simulink model "AUV_velocity_controller"  (R2020b)
settings: Solver=VariableStepAuto  StartTime=0.0  StopTime=400  RelTol=1e-3
libraries: pid_lib x16, robotcorelib x1, dspsigops x1
(part 2 of 2)

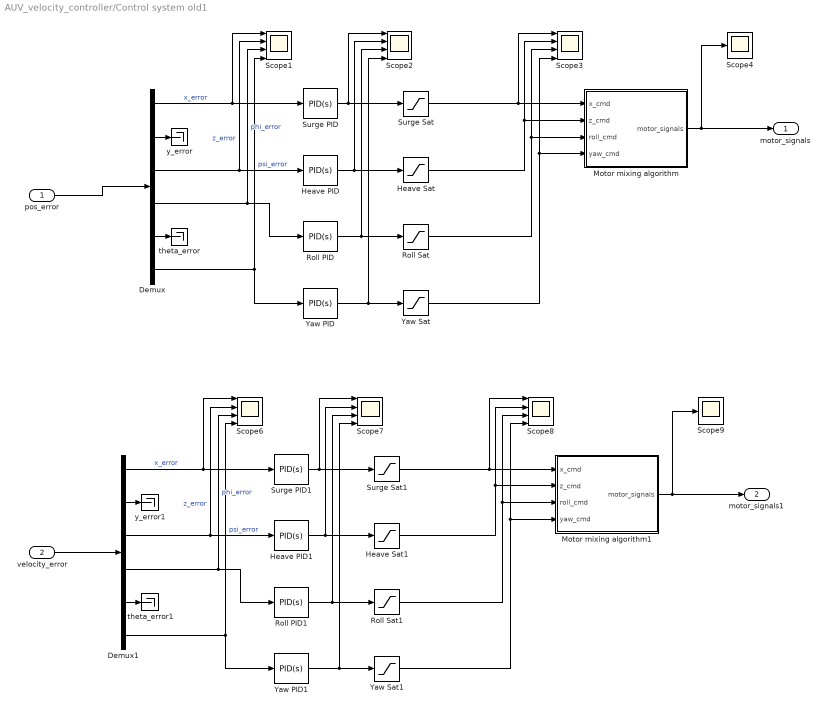
== system AUV_velocity_controller/Control system old1 ==
  pos_error : Inport
  velocity_error : Inport  Port=2
  Demux : Demux  Outputs=6
  Demux1 : Demux  Outputs=6
  Heave PID : pid_lib/PID Controller  Controller=PID  Form=Parallel  TimeDomain=Continuous-time  UseExternalTs=off  SampleTime=-1  IntegratorMethod=Forward Euler  FilterMethod=Forward Euler  ControllerParametersSource=internal  P=5  I=0  D=2  UseFilter=on  N=100  TunerSelectOption=Transfer Function Based (PID Tuner App)  InitialConditionSource=internal  InitialConditionForIntegrator=0  InitialConditionForFilter=0  DifferentiatorICPrevScaledInput=0  ExternalReset=none  TrackingMode=off  Kt=1  LimitOutput=on  SatLimitsSource=internal  UpperSaturationLimit=10  LowerSaturationLimit=-10  LinearizeAsGain=on  AntiWindupMode=clamping  Kb=1  POutMin=[]  POutMax=[]  IOutMin=[]  IOutMax=[]  DOutMin=[]  DOutMax=[]  NOutMin=[]  NOutMax=[]  SumOutMin=[]  SumOutMax=[]  SaturationOutMin=[]  SaturationOutMax=[]  PParamMin=[]  PParamMax=[]  IParamMin=[]  IParamMax=[]  DParamMin=[]  DParamMax=[]  NParamMin=[]  NParamMax=[]  KbParamMin=[]  KbParamMax=[]  KtParamMin=[]  KtParamMax=[]  KbOutMin=[]  KbOutMax=[]  KtOutMin=[]  KtOutMax=[]  IntegratorOutMin=[]  IntegratorOutMax=[]  FilterOutMin=[]  FilterOutMax=[]  SumI1OutMin=[]  SumI1OutMax=[]  SumI2OutMin=[]  SumI2OutMax=[]  SumI3OutMin=[]  SumI3OutMax=[]  SumI4OutMin=[]  SumI4OutMax=[]  SumDOutMin=[]  SumDOutMax=[]  DifferentiatorOutMin=[]  DifferentiatorOutMax=[]  FilterDiffOutCoefMin=[]  FilterDiffOutCoefMax=[]  ReciprocalOutMin=[]  ReciprocalOutMax=[]  SumDenOutMin=[]  SumDenOutMax=[]  SumNumOutMin=[]  SumNumOutMax=[]  DivideOutMin=[]  DivideOutMax=[]  UdiffTsProdOutMin=[]  UdiffTsProdOutMax=[]  NTsProdOutMin=[]  NTsProdOutMax=[]  UintegralTsProdOutMin=[]  UintegralTsProdOutMax=[]  UngainTsProdOutMin=[]  UngainTsProdOutMax=[]  IntegratorContinuousStateAttributes=''  IntegratorStateMustResolveToSignalObject=off  IntegratorRTWStateStorageClass=Auto  FilterContinuousStateAttributes=''  FilterStateMustResolveToSignalObject=off  FilterRTWStateStorageClass=Auto  ParallelPVariant=InternalParameters  IdealPVariant=Disabled  IVariant=InternalParameters  DVariant=InternalParameters  IntegratorVariant=Continuous  SatVariant=Enabled  AWVariant=ContClampingParallel  PCopyVariant=Disabled  TRVariant=Disabled  FdbkBlocksVariant=Forward  IdealPFdbkVariant=Disabled  SatFdbkVariant=Disabled  DerivativeFilterVariant=ContFilter  NVariant=InternalParameters  NCopyVariant=Disabled  FilterICVariant=InternalICsFilter  IntegratorICVariant=InternalICs  ExternalResetVariant=Disabled  TRSumVariant=Passthrough  SumFdbkVariant=Disabled  SumVariant=Sum_PID  TsampFilterVariant=InternalTs  TsampNgainVariant=Passthrough  TsampIntegralVariant=Passthrough  ExternalSaturationOutDataTypeStr=Inherit: Same as second input
  Heave PID1 : pid_lib/PID Controller  Controller=PID  Form=Parallel  TimeDomain=Continuous-time  UseExternalTs=off  SampleTime=-1  IntegratorMethod=Forward Euler  FilterMethod=Forward Euler  ControllerParametersSource=internal  P=5  I=0  D=2  UseFilter=on  N=100  TunerSelectOption=Transfer Function Based (PID Tuner App)  InitialConditionSource=internal  InitialConditionForIntegrator=0  InitialConditionForFilter=0  DifferentiatorICPrevScaledInput=0  ExternalReset=none  TrackingMode=off  Kt=1  LimitOutput=on  SatLimitsSource=internal  UpperSaturationLimit=10  LowerSaturationLimit=-10  LinearizeAsGain=on  AntiWindupMode=clamping  Kb=1  POutMin=[]  POutMax=[]  IOutMin=[]  IOutMax=[]  DOutMin=[]  DOutMax=[]  NOutMin=[]  NOutMax=[]  SumOutMin=[]  SumOutMax=[]  SaturationOutMin=[]  SaturationOutMax=[]  PParamMin=[]  PParamMax=[]  IParamMin=[]  IParamMax=[]  DParamMin=[]  DParamMax=[]  NParamMin=[]  NParamMax=[]  KbParamMin=[]  KbParamMax=[]  KtParamMin=[]  KtParamMax=[]  KbOutMin=[]  KbOutMax=[]  KtOutMin=[]  KtOutMax=[]  IntegratorOutMin=[]  IntegratorOutMax=[]  FilterOutMin=[]  FilterOutMax=[]  SumI1OutMin=[]  SumI1OutMax=[]  SumI2OutMin=[]  SumI2OutMax=[]  SumI3OutMin=[]  SumI3OutMax=[]  SumI4OutMin=[]  SumI4OutMax=[]  SumDOutMin=[]  SumDOutMax=[]  DifferentiatorOutMin=[]  DifferentiatorOutMax=[]  FilterDiffOutCoefMin=[]  FilterDiffOutCoefMax=[]  ReciprocalOutMin=[]  ReciprocalOutMax=[]  SumDenOutMin=[]  SumDenOutMax=[]  SumNumOutMin=[]  SumNumOutMax=[]  DivideOutMin=[]  DivideOutMax=[]  UdiffTsProdOutMin=[]  UdiffTsProdOutMax=[]  NTsProdOutMin=[]  NTsProdOutMax=[]  UintegralTsProdOutMin=[]  UintegralTsProdOutMax=[]  UngainTsProdOutMin=[]  UngainTsProdOutMax=[]  IntegratorContinuousStateAttributes=''  IntegratorStateMustResolveToSignalObject=off  IntegratorRTWStateStorageClass=Auto  FilterContinuousStateAttributes=''  FilterStateMustResolveToSignalObject=off  FilterRTWStateStorageClass=Auto  ParallelPVariant=InternalParameters  IdealPVariant=Disabled  IVariant=InternalParameters  DVariant=InternalParameters  IntegratorVariant=Continuous  SatVariant=Enabled  AWVariant=ContClampingParallel  PCopyVariant=Disabled  TRVariant=Disabled  FdbkBlocksVariant=Forward  IdealPFdbkVariant=Disabled  SatFdbkVariant=Disabled  DerivativeFilterVariant=ContFilter  NVariant=InternalParameters  NCopyVariant=Disabled  FilterICVariant=InternalICsFilter  IntegratorICVariant=InternalICs  ExternalResetVariant=Disabled  TRSumVariant=Passthrough  SumFdbkVariant=Disabled  SumVariant=Sum_PID  TsampFilterVariant=InternalTs  TsampNgainVariant=Passthrough  TsampIntegralVariant=Passthrough  ExternalSaturationOutDataTypeStr=Inherit: Same as second input
  Heave Sat : Saturate  UpperLimit=10  LowerLimit=-10  ZeroCross=off
  Heave Sat1 : Saturate  UpperLimit=10  LowerLimit=-10  ZeroCross=off
  Motor mixing algorithm : MATLAB Function  TreatAsAtomicUnit=on
  Motor mixing algorithm1 : MATLAB Function  TreatAsAtomicUnit=on
  Roll PID : pid_lib/PID Controller  Controller=PID  Form=Parallel  TimeDomain=Continuous-time  UseExternalTs=off  SampleTime=-1  IntegratorMethod=Forward Euler  FilterMethod=Forward Euler  ControllerParametersSource=internal  P=5  I=0  D=2  UseFilter=on  N=100  TunerSelectOption=Transfer Function Based (PID Tuner App)  InitialConditionSource=internal  InitialConditionForIntegrator=0  InitialConditionForFilter=0  DifferentiatorICPrevScaledInput=0  ExternalReset=none  TrackingMode=off  Kt=1  LimitOutput=off  SatLimitsSource=internal  UpperSaturationLimit=inf  LowerSaturationLimit=-inf  LinearizeAsGain=on  AntiWindupMode=none  Kb=1  POutMin=[]  POutMax=[]  IOutMin=[]  IOutMax=[]  DOutMin=[]  DOutMax=[]  NOutMin=[]  NOutMax=[]  SumOutMin=[]  SumOutMax=[]  SaturationOutMin=[]  SaturationOutMax=[]  PParamMin=[]  PParamMax=[]  IParamMin=[]  IParamMax=[]  DParamMin=[]  DParamMax=[]  NParamMin=[]  NParamMax=[]  KbParamMin=[]  KbParamMax=[]  KtParamMin=[]  KtParamMax=[]  KbOutMin=[]  KbOutMax=[]  KtOutMin=[]  KtOutMax=[]  IntegratorOutMin=[]  IntegratorOutMax=[]  FilterOutMin=[]  FilterOutMax=[]  SumI1OutMin=[]  SumI1OutMax=[]  SumI2OutMin=[]  SumI2OutMax=[]  SumI3OutMin=[]  SumI3OutMax=[]  SumI4OutMin=[]  SumI4OutMax=[]  SumDOutMin=[]  SumDOutMax=[]  DifferentiatorOutMin=[]  DifferentiatorOutMax=[]  FilterDiffOutCoefMin=[]  FilterDiffOutCoefMax=[]  ReciprocalOutMin=[]  ReciprocalOutMax=[]  SumDenOutMin=[]  SumDenOutMax=[]  SumNumOutMin=[]  SumNumOutMax=[]  DivideOutMin=[]  DivideOutMax=[]  UdiffTsProdOutMin=[]  UdiffTsProdOutMax=[]  NTsProdOutMin=[]  NTsProdOutMax=[]  UintegralTsProdOutMin=[]  UintegralTsProdOutMax=[]  UngainTsProdOutMin=[]  UngainTsProdOutMax=[]  IntegratorContinuousStateAttributes=''  IntegratorStateMustResolveToSignalObject=off  IntegratorRTWStateStorageClass=Auto  FilterContinuousStateAttributes=''  FilterStateMustResolveToSignalObject=off  FilterRTWStateStorageClass=Auto  ParallelPVariant=InternalParameters  IdealPVariant=Disabled  IVariant=InternalParameters  DVariant=InternalParameters  IntegratorVariant=Continuous  SatVariant=Disabled  AWVariant=Passthrough  PCopyVariant=Disabled  TRVariant=Disabled  FdbkBlocksVariant=Forward  IdealPFdbkVariant=Disabled  SatFdbkVariant=Disabled  DerivativeFilterVariant=ContFilter  NVariant=InternalParameters  NCopyVariant=Disabled  FilterICVariant=InternalICsFilter  IntegratorICVariant=InternalICs  ExternalResetVariant=Disabled  TRSumVariant=Passthrough  SumFdbkVariant=Disabled  SumVariant=Sum_PID  TsampFilterVariant=InternalTs  TsampNgainVariant=Passthrough  TsampIntegralVariant=Passthrough  ExternalSaturationOutDataTypeStr=Inherit: Same as second input
  Roll PID1 : pid_lib/PID Controller  Controller=PID  Form=Parallel  TimeDomain=Continuous-time  UseExternalTs=off  SampleTime=-1  IntegratorMethod=Forward Euler  FilterMethod=Forward Euler  ControllerParametersSource=internal  P=5  I=0  D=2  UseFilter=on  N=100  TunerSelectOption=Transfer Function Based (PID Tuner App)  InitialConditionSource=internal  InitialConditionForIntegrator=0  InitialConditionForFilter=0  DifferentiatorICPrevScaledInput=0  ExternalReset=none  TrackingMode=off  Kt=1  LimitOutput=off  SatLimitsSource=internal  UpperSaturationLimit=inf  LowerSaturationLimit=-inf  LinearizeAsGain=on  AntiWindupMode=none  Kb=1  POutMin=[]  POutMax=[]  IOutMin=[]  IOutMax=[]  DOutMin=[]  DOutMax=[]  NOutMin=[]  NOutMax=[]  SumOutMin=[]  SumOutMax=[]  SaturationOutMin=[]  SaturationOutMax=[]  PParamMin=[]  PParamMax=[]  IParamMin=[]  IParamMax=[]  DParamMin=[]  DParamMax=[]  NParamMin=[]  NParamMax=[]  KbParamMin=[]  KbParamMax=[]  KtParamMin=[]  KtParamMax=[]  KbOutMin=[]  KbOutMax=[]  KtOutMin=[]  KtOutMax=[]  IntegratorOutMin=[]  IntegratorOutMax=[]  FilterOutMin=[]  FilterOutMax=[]  SumI1OutMin=[]  SumI1OutMax=[]  SumI2OutMin=[]  SumI2OutMax=[]  SumI3OutMin=[]  SumI3OutMax=[]  SumI4OutMin=[]  SumI4OutMax=[]  SumDOutMin=[]  SumDOutMax=[]  DifferentiatorOutMin=[]  DifferentiatorOutMax=[]  FilterDiffOutCoefMin=[]  FilterDiffOutCoefMax=[]  ReciprocalOutMin=[]  ReciprocalOutMax=[]  SumDenOutMin=[]  SumDenOutMax=[]  SumNumOutMin=[]  SumNumOutMax=[]  DivideOutMin=[]  DivideOutMax=[]  UdiffTsProdOutMin=[]  UdiffTsProdOutMax=[]  NTsProdOutMin=[]  NTsProdOutMax=[]  UintegralTsProdOutMin=[]  UintegralTsProdOutMax=[]  UngainTsProdOutMin=[]  UngainTsProdOutMax=[]  IntegratorContinuousStateAttributes=''  IntegratorStateMustResolveToSignalObject=off  IntegratorRTWStateStorageClass=Auto  FilterContinuousStateAttributes=''  FilterStateMustResolveToSignalObject=off  FilterRTWStateStorageClass=Auto  ParallelPVariant=InternalParameters  IdealPVariant=Disabled  IVariant=InternalParameters  DVariant=InternalParameters  IntegratorVariant=Continuous  SatVariant=Disabled  AWVariant=Passthrough  PCopyVariant=Disabled  TRVariant=Disabled  FdbkBlocksVariant=Forward  IdealPFdbkVariant=Disabled  SatFdbkVariant=Disabled  DerivativeFilterVariant=ContFilter  NVariant=InternalParameters  NCopyVariant=Disabled  FilterICVariant=InternalICsFilter  IntegratorICVariant=InternalICs  ExternalResetVariant=Disabled  TRSumVariant=Passthrough  SumFdbkVariant=Disabled  SumVariant=Sum_PID  TsampFilterVariant=InternalTs  TsampNgainVariant=Passthrough  TsampIntegralVariant=Passthrough  ExternalSaturationOutDataTypeStr=Inherit: Same as second input
  Roll Sat : Saturate  UpperLimit=10  LowerLimit=-10  ZeroCross=off
  Roll Sat1 : Saturate  UpperLimit=10  LowerLimit=-10  ZeroCross=off
  Scope{1..3,6..8} (6 alike) : Scope  NumInputPorts=4
  Scope4 : Scope
  Scope9 : Scope
  Surge PID : pid_lib/PID Controller  Controller=PID  Form=Parallel  TimeDomain=Continuous-time  UseExternalTs=off  SampleTime=-1  IntegratorMethod=Forward Euler  FilterMethod=Forward Euler  ControllerParametersSource=internal  P=5  I=0  D=2  UseFilter=on  N=100  TunerSelectOption=Transfer Function Based (PID Tuner App)  InitialConditionSource=internal  InitialConditionForIntegrator=0  InitialConditionForFilter=0  DifferentiatorICPrevScaledInput=0  ExternalReset=none  TrackingMode=off  Kt=1  LimitOutput=on  SatLimitsSource=internal  UpperSaturationLimit=10  LowerSaturationLimit=-10  LinearizeAsGain=on  AntiWindupMode=clamping  Kb=1  POutMin=[]  POutMax=[]  IOutMin=[]  IOutMax=[]  DOutMin=[]  DOutMax=[]  NOutMin=[]  NOutMax=[]  SumOutMin=[]  SumOutMax=[]  SaturationOutMin=[]  SaturationOutMax=[]  PParamMin=[]  PParamMax=[]  IParamMin=[]  IParamMax=[]  DParamMin=[]  DParamMax=[]  NParamMin=[]  NParamMax=[]  KbParamMin=[]  KbParamMax=[]  KtParamMin=[]  KtParamMax=[]  KbOutMin=[]  KbOutMax=[]  KtOutMin=[]  KtOutMax=[]  IntegratorOutMin=[]  IntegratorOutMax=[]  FilterOutMin=[]  FilterOutMax=[]  SumI1OutMin=[]  SumI1OutMax=[]  SumI2OutMin=[]  SumI2OutMax=[]  SumI3OutMin=[]  SumI3OutMax=[]  SumI4OutMin=[]  SumI4OutMax=[]  SumDOutMin=[]  SumDOutMax=[]  DifferentiatorOutMin=[]  DifferentiatorOutMax=[]  FilterDiffOutCoefMin=[]  FilterDiffOutCoefMax=[]  ReciprocalOutMin=[]  ReciprocalOutMax=[]  SumDenOutMin=[]  SumDenOutMax=[]  SumNumOutMin=[]  SumNumOutMax=[]  DivideOutMin=[]  DivideOutMax=[]  UdiffTsProdOutMin=[]  UdiffTsProdOutMax=[]  NTsProdOutMin=[]  NTsProdOutMax=[]  UintegralTsProdOutMin=[]  UintegralTsProdOutMax=[]  UngainTsProdOutMin=[]  UngainTsProdOutMax=[]  IntegratorContinuousStateAttributes=''  IntegratorStateMustResolveToSignalObject=off  IntegratorRTWStateStorageClass=Auto  FilterContinuousStateAttributes=''  FilterStateMustResolveToSignalObject=off  FilterRTWStateStorageClass=Auto  ParallelPVariant=InternalParameters  IdealPVariant=Disabled  IVariant=InternalParameters  DVariant=InternalParameters  IntegratorVariant=Continuous  SatVariant=Enabled  AWVariant=ContClampingParallel  PCopyVariant=Disabled  TRVariant=Disabled  FdbkBlocksVariant=Forward  IdealPFdbkVariant=Disabled  SatFdbkVariant=Disabled  DerivativeFilterVariant=ContFilter  NVariant=InternalParameters  NCopyVariant=Disabled  FilterICVariant=InternalICsFilter  IntegratorICVariant=InternalICs  ExternalResetVariant=Disabled  TRSumVariant=Passthrough  SumFdbkVariant=Disabled  SumVariant=Sum_PID  TsampFilterVariant=InternalTs  TsampNgainVariant=Passthrough  TsampIntegralVariant=Passthrough  ExternalSaturationOutDataTypeStr=Inherit: Same as second input
  Surge PID1 : pid_lib/PID Controller  Controller=PID  Form=Parallel  TimeDomain=Continuous-time  UseExternalTs=off  SampleTime=-1  IntegratorMethod=Forward Euler  FilterMethod=Forward Euler  ControllerParametersSource=internal  P=5  I=0  D=2  UseFilter=on  N=100  TunerSelectOption=Transfer Function Based (PID Tuner App)  InitialConditionSource=internal  InitialConditionForIntegrator=0  InitialConditionForFilter=0  DifferentiatorICPrevScaledInput=0  ExternalReset=none  TrackingMode=off  Kt=1  LimitOutput=on  SatLimitsSource=internal  UpperSaturationLimit=10  LowerSaturationLimit=-10  LinearizeAsGain=on  AntiWindupMode=clamping  Kb=1  POutMin=[]  POutMax=[]  IOutMin=[]  IOutMax=[]  DOutMin=[]  DOutMax=[]  NOutMin=[]  NOutMax=[]  SumOutMin=[]  SumOutMax=[]  SaturationOutMin=[]  SaturationOutMax=[]  PParamMin=[]  PParamMax=[]  IParamMin=[]  IParamMax=[]  DParamMin=[]  DParamMax=[]  NParamMin=[]  NParamMax=[]  KbParamMin=[]  KbParamMax=[]  KtParamMin=[]  KtParamMax=[]  KbOutMin=[]  KbOutMax=[]  KtOutMin=[]  KtOutMax=[]  IntegratorOutMin=[]  IntegratorOutMax=[]  FilterOutMin=[]  FilterOutMax=[]  SumI1OutMin=[]  SumI1OutMax=[]  SumI2OutMin=[]  SumI2OutMax=[]  SumI3OutMin=[]  SumI3OutMax=[]  SumI4OutMin=[]  SumI4OutMax=[]  SumDOutMin=[]  SumDOutMax=[]  DifferentiatorOutMin=[]  DifferentiatorOutMax=[]  FilterDiffOutCoefMin=[]  FilterDiffOutCoefMax=[]  ReciprocalOutMin=[]  ReciprocalOutMax=[]  SumDenOutMin=[]  SumDenOutMax=[]  SumNumOutMin=[]  SumNumOutMax=[]  DivideOutMin=[]  DivideOutMax=[]  UdiffTsProdOutMin=[]  UdiffTsProdOutMax=[]  NTsProdOutMin=[]  NTsProdOutMax=[]  UintegralTsProdOutMin=[]  UintegralTsProdOutMax=[]  UngainTsProdOutMin=[]  UngainTsProdOutMax=[]  IntegratorContinuousStateAttributes=''  IntegratorStateMustResolveToSignalObject=off  IntegratorRTWStateStorageClass=Auto  FilterContinuousStateAttributes=''  FilterStateMustResolveToSignalObject=off  FilterRTWStateStorageClass=Auto  ParallelPVariant=InternalParameters  IdealPVariant=Disabled  IVariant=InternalParameters  DVariant=InternalParameters  IntegratorVariant=Continuous  SatVariant=Enabled  AWVariant=ContClampingParallel  PCopyVariant=Disabled  TRVariant=Disabled  FdbkBlocksVariant=Forward  IdealPFdbkVariant=Disabled  SatFdbkVariant=Disabled  DerivativeFilterVariant=ContFilter  NVariant=InternalParameters  NCopyVariant=Disabled  FilterICVariant=InternalICsFilter  IntegratorICVariant=InternalICs  ExternalResetVariant=Disabled  TRSumVariant=Passthrough  SumFdbkVariant=Disabled  SumVariant=Sum_PID  TsampFilterVariant=InternalTs  TsampNgainVariant=Passthrough  TsampIntegralVariant=Passthrough  ExternalSaturationOutDataTypeStr=Inherit: Same as second input
  Surge Sat : Saturate  UpperLimit=10  LowerLimit=-10  ZeroCross=off
  Surge Sat1 : Saturate  UpperLimit=10  LowerLimit=-10  ZeroCross=off
  Yaw PID : pid_lib/PID Controller  Controller=PID  Form=Parallel  TimeDomain=Continuous-time  UseExternalTs=off  SampleTime=-1  IntegratorMethod=Forward Euler  FilterMethod=Forward Euler  ControllerParametersSource=internal  P=5  I=0  D=2  UseFilter=on  N=100  TunerSelectOption=Transfer Function Based (PID Tuner App)  InitialConditionSource=internal  InitialConditionForIntegrator=0  InitialConditionForFilter=0  DifferentiatorICPrevScaledInput=0  ExternalReset=none  TrackingMode=off  Kt=1  LimitOutput=off  SatLimitsSource=internal  UpperSaturationLimit=inf  LowerSaturationLimit=-inf  LinearizeAsGain=on  AntiWindupMode=none  Kb=1  POutMin=[]  POutMax=[]  IOutMin=[]  IOutMax=[]  DOutMin=[]  DOutMax=[]  NOutMin=[]  NOutMax=[]  SumOutMin=[]  SumOutMax=[]  SaturationOutMin=[]  SaturationOutMax=[]  PParamMin=[]  PParamMax=[]  IParamMin=[]  IParamMax=[]  DParamMin=[]  DParamMax=[]  NParamMin=[]  NParamMax=[]  KbParamMin=[]  KbParamMax=[]  KtParamMin=[]  KtParamMax=[]  KbOutMin=[]  KbOutMax=[]  KtOutMin=[]  KtOutMax=[]  IntegratorOutMin=[]  IntegratorOutMax=[]  FilterOutMin=[]  FilterOutMax=[]  SumI1OutMin=[]  SumI1OutMax=[]  SumI2OutMin=[]  SumI2OutMax=[]  SumI3OutMin=[]  SumI3OutMax=[]  SumI4OutMin=[]  SumI4OutMax=[]  SumDOutMin=[]  SumDOutMax=[]  DifferentiatorOutMin=[]  DifferentiatorOutMax=[]  FilterDiffOutCoefMin=[]  FilterDiffOutCoefMax=[]  ReciprocalOutMin=[]  ReciprocalOutMax=[]  SumDenOutMin=[]  SumDenOutMax=[]  SumNumOutMin=[]  SumNumOutMax=[]  DivideOutMin=[]  DivideOutMax=[]  UdiffTsProdOutMin=[]  UdiffTsProdOutMax=[]  NTsProdOutMin=[]  NTsProdOutMax=[]  UintegralTsProdOutMin=[]  UintegralTsProdOutMax=[]  UngainTsProdOutMin=[]  UngainTsProdOutMax=[]  IntegratorContinuousStateAttributes=''  IntegratorStateMustResolveToSignalObject=off  IntegratorRTWStateStorageClass=Auto  FilterContinuousStateAttributes=''  FilterStateMustResolveToSignalObject=off  FilterRTWStateStorageClass=Auto  ParallelPVariant=InternalParameters  IdealPVariant=Disabled  IVariant=InternalParameters  DVariant=InternalParameters  IntegratorVariant=Continuous  SatVariant=Disabled  AWVariant=Passthrough  PCopyVariant=Disabled  TRVariant=Disabled  FdbkBlocksVariant=Forward  IdealPFdbkVariant=Disabled  SatFdbkVariant=Disabled  DerivativeFilterVariant=ContFilter  NVariant=InternalParameters  NCopyVariant=Disabled  FilterICVariant=InternalICsFilter  IntegratorICVariant=InternalICs  ExternalResetVariant=Disabled  TRSumVariant=Passthrough  SumFdbkVariant=Disabled  SumVariant=Sum_PID  TsampFilterVariant=InternalTs  TsampNgainVariant=Passthrough  TsampIntegralVariant=Passthrough  ExternalSaturationOutDataTypeStr=Inherit: Same as second input
  Yaw PID1 : pid_lib/PID Controller  Controller=PID  Form=Parallel  TimeDomain=Continuous-time  UseExternalTs=off  SampleTime=-1  IntegratorMethod=Forward Euler  FilterMethod=Forward Euler  ControllerParametersSource=internal  P=5  I=0  D=2  UseFilter=on  N=100  TunerSelectOption=Transfer Function Based (PID Tuner App)  InitialConditionSource=internal  InitialConditionForIntegrator=0  InitialConditionForFilter=0  DifferentiatorICPrevScaledInput=0  ExternalReset=none  TrackingMode=off  Kt=1  LimitOutput=off  SatLimitsSource=internal  UpperSaturationLimit=inf  LowerSaturationLimit=-inf  LinearizeAsGain=on  AntiWindupMode=none  Kb=1  POutMin=[]  POutMax=[]  IOutMin=[]  IOutMax=[]  DOutMin=[]  DOutMax=[]  NOutMin=[]  NOutMax=[]  SumOutMin=[]  SumOutMax=[]  SaturationOutMin=[]  SaturationOutMax=[]  PParamMin=[]  PParamMax=[]  IParamMin=[]  IParamMax=[]  DParamMin=[]  DParamMax=[]  NParamMin=[]  NParamMax=[]  KbParamMin=[]  KbParamMax=[]  KtParamMin=[]  KtParamMax=[]  KbOutMin=[]  KbOutMax=[]  KtOutMin=[]  KtOutMax=[]  IntegratorOutMin=[]  IntegratorOutMax=[]  FilterOutMin=[]  FilterOutMax=[]  SumI1OutMin=[]  SumI1OutMax=[]  SumI2OutMin=[]  SumI2OutMax=[]  SumI3OutMin=[]  SumI3OutMax=[]  SumI4OutMin=[]  SumI4OutMax=[]  SumDOutMin=[]  SumDOutMax=[]  DifferentiatorOutMin=[]  DifferentiatorOutMax=[]  FilterDiffOutCoefMin=[]  FilterDiffOutCoefMax=[]  ReciprocalOutMin=[]  ReciprocalOutMax=[]  SumDenOutMin=[]  SumDenOutMax=[]  SumNumOutMin=[]  SumNumOutMax=[]  DivideOutMin=[]  DivideOutMax=[]  UdiffTsProdOutMin=[]  UdiffTsProdOutMax=[]  NTsProdOutMin=[]  NTsProdOutMax=[]  UintegralTsProdOutMin=[]  UintegralTsProdOutMax=[]  UngainTsProdOutMin=[]  UngainTsProdOutMax=[]  IntegratorContinuousStateAttributes=''  IntegratorStateMustResolveToSignalObject=off  IntegratorRTWStateStorageClass=Auto  FilterContinuousStateAttributes=''  FilterStateMustResolveToSignalObject=off  FilterRTWStateStorageClass=Auto  ParallelPVariant=InternalParameters  IdealPVariant=Disabled  IVariant=InternalParameters  DVariant=InternalParameters  IntegratorVariant=Continuous  SatVariant=Disabled  AWVariant=Passthrough  PCopyVariant=Disabled  TRVariant=Disabled  FdbkBlocksVariant=Forward  IdealPFdbkVariant=Disabled  SatFdbkVariant=Disabled  DerivativeFilterVariant=ContFilter  NVariant=InternalParameters  NCopyVariant=Disabled  FilterICVariant=InternalICsFilter  IntegratorICVariant=InternalICs  ExternalResetVariant=Disabled  TRSumVariant=Passthrough  SumFdbkVariant=Disabled  SumVariant=Sum_PID  TsampFilterVariant=InternalTs  TsampNgainVariant=Passthrough  TsampIntegralVariant=Passthrough  ExternalSaturationOutDataTypeStr=Inherit: Same as second input
  Yaw Sat : Saturate  UpperLimit=10  LowerLimit=-10  ZeroCross=off
  Yaw Sat1 : Saturate  UpperLimit=10  LowerLimit=-10  ZeroCross=off
  theta_error : Terminator
  theta_error1 : Terminator
  y_error : Terminator
  y_error1 : Terminator
  motor_signals : Outport
  motor_signals1 : Outport  Port=2
  wires:
  Demux/4 -> Scope1/3, Roll PID/1  "phi_error"
  Demux/3 -> Scope1/2, Heave PID/1  "z_error"
  Demux/6 -> Scope1/4, Yaw PID/1  "psi_error"
  Demux/1 -> Scope1/1, Surge PID/1  "x_error"
  pos_error/1 -> Demux/1
  Demux/5 -> theta_error/1
  Demux/2 -> y_error/1
  Yaw PID/1 -> Scope2/4, Yaw Sat/1
  Roll PID/1 -> Roll Sat/1, Scope2/3
  Heave PID/1 -> Heave Sat/1, Scope2/2
  Surge PID/1 -> Surge Sat/1, Scope2/1
  Surge Sat/1 -> Scope3/1, Motor mixing algorithm/1(x_cmd)
  Heave Sat/1 -> Scope3/2, Motor mixing algorithm/2(z_cmd)
  Yaw Sat/1 -> Motor mixing algorithm/4(yaw_cmd), Scope3/4
  Roll Sat/1 -> Scope3/3, Motor mixing algorithm/3(roll_cmd)
  Motor mixing algorithm/1(motor_signals) -> motor_signals/1, Scope4/1
  Demux1/4 -> Scope6/3, Roll PID1/1  "phi_error"
  Surge Sat1/1 -> Scope8/1, Motor mixing algorithm1/1(x_cmd)
  Demux1/5 -> theta_error1/1
  Heave PID1/1 -> Heave Sat1/1, Scope7/2
  Demux1/6 -> Scope6/4, Yaw PID1/1  "psi_error"
  Demux1/2 -> y_error1/1
  Demux1/3 -> Scope6/2, Heave PID1/1  "z_error"
  velocity_error/1 -> Demux1/1
  Yaw PID1/1 -> Scope7/4, Yaw Sat1/1
  Roll Sat1/1 -> Scope8/3, Motor mixing algorithm1/3(roll_cmd)
  Surge PID1/1 -> Surge Sat1/1, Scope7/1
  Roll PID1/1 -> Roll Sat1/1, Scope7/3
  Demux1/1 -> Scope6/1, Surge PID1/1  "x_error"
  Yaw Sat1/1 -> Motor mixing algorithm1/4(yaw_cmd), Scope8/4
  Motor mixing algorithm1/1(motor_signals) -> motor_signals1/1, Scope9/1
  Heave Sat1/1 -> Scope8/2, Motor mixing algorithm1/2(z_cmd)

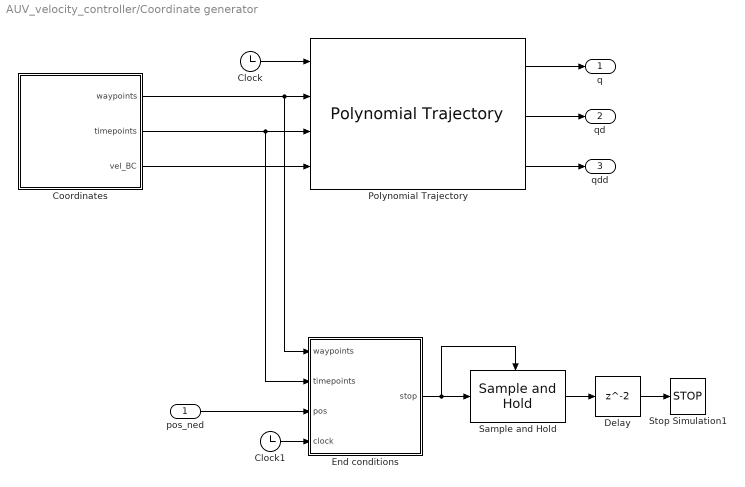
== system AUV_velocity_controller/Coordinate generator ==
  pos_ned : Inport
  Clock : Clock
  Clock1 : Clock
  Coordinates : MATLAB Function  TreatAsAtomicUnit=on
  Delay : Delay  InputProcessing=Columns as channels (frame based)
  End conditions : MATLAB Function  TreatAsAtomicUnit=on
  Polynomial Trajectory : robotcorelib/Polynomial Trajectory  WaypointSource=External  Waypoints=[ 0, 2, 1, 5, 0; -1, 3, 1, 4, 4 ]  TimePoints=[ 0, 1, 2, 3, 4 ]  TimeInterval=[ 1, 4 ]  Method=Cubic Polynomial  ParameterSource=External  VelocityBoundaryCondition=zeros( 2, 5 )  AccelerationBoundaryCondition=zeros( 2, 5 )  SimulateUsing=Interpreted execution
  Sample and Hold : dspsigops/Sample and Hold  trig=Rising edge  initCond=0  latchinput=off
  Stop Simulation1 : Stop
  q : Outport
  qd : Outport  Port=2
  qdd : Outport  Port=3
  wires:
  Coordinates/3(vel_BC) -> Polynomial Trajectory/4
  Polynomial Trajectory/1 -> q/1
  Polynomial Trajectory/3 -> qdd/1
  Coordinates/2(timepoints) -> Polynomial Trajectory/3, End conditions/2(timepoints)
  Polynomial Trajectory/2 -> qd/1
  Coordinates/1(waypoints) -> End conditions/1(waypoints), Polynomial Trajectory/2
  Clock/1 -> Polynomial Trajectory/1
  Clock1/1 -> End conditions/4(clock)
  pos_ned/1 -> End conditions/3(pos)
  Delay/1 -> Stop Simulation1/1
  End conditions/1(stop) -> Sample and Hold/Trigger, Sample and Hold/1
  Sample and Hold/1 -> Delay/1

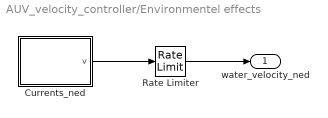
== system AUV_velocity_controller/Environmentel effects ==
  Currents_ned : MATLAB Function  TreatAsAtomicUnit=on
  Rate Limiter : RateLimiter  RisingSlewLimit=10  FallingSlewLimit=-10  SampleTimeMode=inherited
  water_velocity_ned : Outport
  wires:
  Currents_ned/1(v) -> Rate Limiter/1
  Rate Limiter/1 -> water_velocity_ned/1

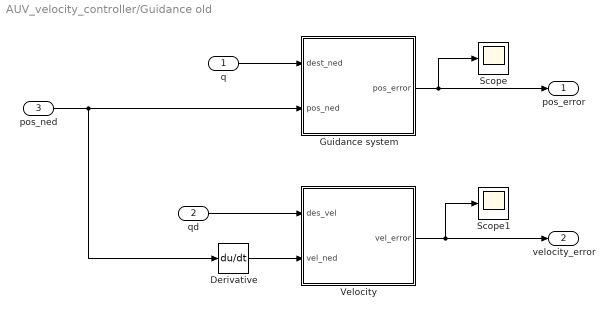
== system AUV_velocity_controller/Guidance old ==
  q : Inport
  qd : Inport  Port=2
  pos_ned : Inport  Port=3
  Derivative : Derivative
  Guidance system : MATLAB Function  TreatAsAtomicUnit=on
  Scope : Scope
  Scope1 : Scope
  "Velocity " : MATLAB Function  TreatAsAtomicUnit=on
  pos_error : Outport
  velocity_error : Outport  Port=2
  wires:
  q/1 -> Guidance system/1(dest_ned)
  Guidance system/1(pos_error) -> pos_error/1, Scope/1
  pos_ned/1 -> Derivative/1, Guidance system/2(pos_ned)
  "Velocity "/1(vel_error) -> Scope1/1, velocity_error/1
  Derivative/1 -> "Velocity "/2(vel_ned)
  qd/1 -> "Velocity "/1(des_vel)

== matlab function AUV_velocity_controller/Coordinate generator/Coordinates ==
  data: waypoints output; timepoints output; vel_BC output
function [waypoints, timepoints, vel_BC] = fcn()

    avg_speed = 0.5; % m/s
    
    waypoints = [
    0, 10, 10, -10, -10,  10, 0;
    0,  0, 10,  10, -10, -10, 0;
    0,  0, 5,   10,   0,   0, 0; 
    ];
    
    [~, n] = size(waypoints);
    timepoints = zeros(1, n);
    for i = 2:n
        distance = norm(waypoints(1:3, i) - waypoints(1:3, i-1));
        timepoints(1, i) = timepoints(1, i-1) + distance/avg_speed;
    end
   
    vel_BC = zeros(size(waypoints));
    for i = 2:n-1
        direction = waypoints(1:3, i+1) - waypoints(1:3, i-1);
        unit_d = direction / norm(direction);
        vel_BC(1:3, i) = avg_speed * unit_d;
    end
end

== matlab function AUV_velocity_controller/Control system old/Motor mixing algorithm ==
  data: x_cmd input; motor_signals output size=[1, 4]; z_cmd input; roll_cmd input; yaw_cmd input
function motor_signals = fcn(x_cmd, z_cmd, roll_cmd, yaw_cmd)

front_right_motor = -z_cmd - roll_cmd;
front_left_motor = -z_cmd + roll_cmd;
back_right_motor = x_cmd - yaw_cmd;
back_left_motor = x_cmd + yaw_cmd;

motor_signals = [front_right_motor, front_left_motor, back_right_motor, back_left_motor];
end

== matlab function AUV_velocity_controller/Control system old1/Motor mixing algorithm1 ==
  data: x_cmd input; motor_signals output size=[1, 4]; z_cmd input; roll_cmd input; yaw_cmd input
function motor_signals = fcn(x_cmd, z_cmd, roll_cmd, yaw_cmd)

front_right_motor = -z_cmd - roll_cmd;
front_left_motor = -z_cmd + roll_cmd;
back_right_motor = x_cmd - yaw_cmd;
back_left_motor = x_cmd + yaw_cmd;

motor_signals = [front_right_motor, front_left_motor, back_right_motor, back_left_motor];
end

== matlab function AUV_velocity_controller/3D scope/3D plot ==
  data: traj input; plot output; pos input
function plot = fcn(traj, pos)
 plot = [traj(2); traj(1); -traj(3); pos(2); pos(1); -pos(3)];

== matlab function AUV_velocity_controller/Guidance old/Velocity  ==
  data: des_vel input; vel_error output; vel_ned input
function vel_error = fcn(des_vel, vel_ned)
    % note that x is north, y is east and z is down    
    N_error = des_vel(1)-vel_ned(1);
    E_error = des_vel(2)-vel_ned(2);
    D_error = des_vel(3)-vel_ned(3);

    current_heading = vel_ned(6);
    desired_heading = atan2(E_error, N_error);

    % convert to body axis
    x_error = max([-1, N_error*cos(current_heading)+E_error*sin(current_heading)]);
    y_error = 0;
    z_error = D_error;

    roll_error = 0;
    pitch_error = 0;
    yaw_error = desired_heading - current_heading;
    
    while roll_error > pi
        roll_error = roll_error - 2*pi;
    end
    while roll_error < -pi
        roll_error = roll_error + 2*pi;
    end

    while yaw_error > pi
        yaw_error = yaw_error - 2*pi;
    end
    while yaw_error < -pi
        yaw_error = yaw_error + 2*pi;
    end
    
    % Scale x_error down when yaw_error is high 
%      k_angle = yaw_error*3;
%      if k_angle > pi || k_angle < -pi
%          k_angle = pi;
%      end
%       
%      k = 0.5*cos(k_angle)+0.5;
%      x_error = x_error*k;
    
    % Prevent turning if XY destination is nearby
%      arrival_error = 0.2;
%      NE_error = abs(N_error) + abs(E_error);
%      if NE_error < arrival_error
%          x_error = 0;
%          yaw_error = 0; % to prevent circling
%      end
%      if abs(D_error) < arrival_error
%          z_error = 0;
%      end
    
    vel_error = [x_error; y_error; z_error; roll_error; pitch_error; yaw_error];
end

== matlab function AUV_velocity_controller/Environmentel effects/Currents_ned ==
  data: v output
function v = fcn()
    % currents are irrotational
    v = [0; 0; 0];
end

== matlab function AUV_velocity_controller/AUV Dynamics/Motor Forces ==
  data: F_control output size=6; motor_signals input
function F_control = fcn(motor_signals)
% x, y and z axis relates to local front (bow), starboard and down
% directions
% phi, theta and psi represents roll, pitch and yaw respectivly

% assuming that the force produced by each motor is proportonal to the
% signal voltage

thrust_constant = 1;
roll_constant = 1;
yaw_constant = 1;

FrontRight_m = motor_signals(1);
FrontLeft_m = motor_signals(2);
BackRight_m = motor_signals(3);
BackLeft_m = motor_signals(4);

F_control = [thrust_constant*(BackRight_m+BackLeft_m); 
      0;                                            % AUV cannot move in y direction
      -thrust_constant*(FrontRight_m+FrontLeft_m);  % positive z is downward 
      roll_constant*(FrontLeft_m-FrontRight_m);     % positive rotation is clockwise
      0;                                            % AUV cannot pitch 
      yaw_constant*(BackLeft_m-BackRight_m);
];

== matlab function AUV_velocity_controller/AUV Dynamics/AUV Kinematics ==
  data: v_body input; ned_pos input; v_ned output
function v_ned = fcn(v_body, ned_pos)

% calculate Jacobian using MSS toolbox function
    [J, ~, ~] = eulerang(ned_pos(4), ned_pos(5), ned_pos(6)); 
    v_ned = J * v_body;
end

== matlab function AUV_velocity_controller/Coordinate generator/End conditions ==
  data: waypoints input; timepoints input; pos input; clock input; stop output
function stop = fcn(waypoints, timepoints, pos, clock)

    final_n_error = abs(pos(1) - waypoints(1, end));
    final_e_error = abs(pos(2) - waypoints(2, end));
    final_d_error = abs(pos(3) - waypoints(3, end));
    final_pos_error = final_n_error + final_e_error + final_d_error;
    acceptance_radius = 0.5;

    if clock > timepoints(1, end) && final_pos_error < acceptance_radius
        stop = 1;
    else
        stop = 0;
    end
end

== matlab function AUV_velocity_controller/AUV Dynamics/AUV dynamic model ==
  data: F_ctrl input; Cv output; Dv output; a_body output size=6; v_c input; v input
function [Cv, Dv, a_body] = fcn(F_ctrl, v_c, v)

v_r = v - v_c;
[M, C, D, g] = AUV_dynamic_model(v_r);    

% For output scope
Cv = C*v_r;
Dv = D*v_r;

a_body = M\(F_ctrl - C*v_r - D*v_r - g);

== matlab function AUV_velocity_controller/Guidance old/Guidance system ==
  data: dest_ned input; pos_error output; pos_ned input
function pos_error = fcn(dest_ned, pos_ned)
    % note that x is north, y is east and z is down    
    N_error = dest_ned(1)-pos_ned(1);
    E_error = dest_ned(2)-pos_ned(2);
    D_error = dest_ned(3)-pos_ned(3);

    current_heading = pos_ned(6);
    desired_heading = atan2(E_error, N_error);

    % convert to body axis
    x_error = max([-1, N_error*cos(current_heading)+E_error*sin(current_heading)]);
    y_error = 0;
    z_error = D_error;

    roll_error = 0;
    pitch_error = 0;
    yaw_error = desired_heading - current_heading;
    
    while roll_error > pi
        roll_error = roll_error - 2*pi;
    end
    while roll_error < -pi
        roll_error = roll_error + 2*pi;
    end

    while yaw_error > pi
        yaw_error = yaw_error - 2*pi;
    end
    while yaw_error < -pi
        yaw_error = yaw_error + 2*pi;
    end
    
    % Scale x_error down when yaw_error is high 
     k_angle = yaw_error*3;
     if k_angle > pi || k_angle < -pi
         k_angle = pi;
     end
      
     k = 0.5*cos(k_angle)+0.5;
     x_error = x_error*k;
    
    % Prevent turning if XY destination is nearby
%      arrival_error = 0.2;
%      NE_error = abs(N_error) + abs(E_error);
%      if NE_error < arrival_error
%          x_error = 0;
%          yaw_error = 0; % to prevent circling
%      end
%      if abs(D_error) < arrival_error
%          z_error = 0;
%      end
    
    pos_error = [x_error; y_error; z_error; roll_error; pitch_error; yaw_error];
end

== matlab function AUV_velocity_controller/AUV Dynamics/Environment Kinematics ==
  data: water_velocity_ned input; water_velocity_body output size=6; pos_ned input
function water_velocity_body = fcn(water_velocity_ned, pos_ned)
    euler_ang = rotateZYX(pos_ned(4), pos_ned(5), pos_ned(6));
    w_v =  euler_ang * water_velocity_ned;
    water_velocity_body = [w_v(1); w_v(2); w_v(3); 0; 0; 0];
end

== matlab function AUV_velocity_controller/Control system old1/Motor mixing algorithm ==
  data: x_cmd input; motor_signals output size=[1, 4]; z_cmd input; roll_cmd input; yaw_cmd input
function motor_signals = fcn(x_cmd, z_cmd, roll_cmd, yaw_cmd)

front_right_motor = -z_cmd - roll_cmd;
front_left_motor = -z_cmd + roll_cmd;
back_right_motor = x_cmd - yaw_cmd;
back_left_motor = x_cmd + yaw_cmd;

motor_signals = [front_right_motor, front_left_motor, back_right_motor, back_left_motor];
end
